simulink model "simulation_environment"  (R2018b)
settings: Solver=VariableStepAuto  StartTime=0.0  StopTime=50  RelTol=1e-3
libraries: follow_the_leader_library x3
settings Model: Creator=martin  LastModifiedBy=martin

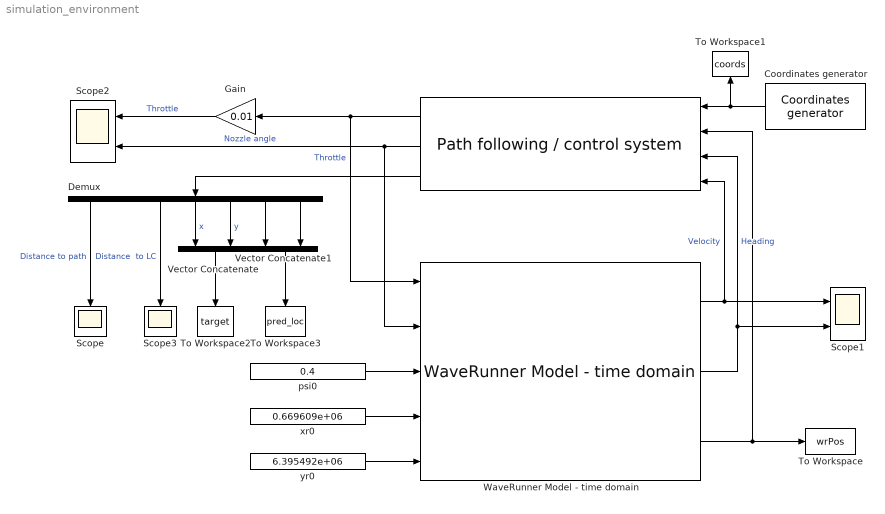
== system simulation_environment ==
  " " : follow_the_leader_library/Path following // control system  dt=2  g_Kp=4  g_Tf=5  g_Kd=0  g_Ki=5  g_max=100  g_min=0  n_Kp=-1  n_Tf=1  n_Kd=-100  n_Ki=0  n_max=18 * pi / 180  n_min=-18 * pi / 180
      settings: SourceProductName=Follow the leader
  Coordinates generator : follow_the_leader_library/Coordinates generator  fname=test3.txt  steptime=0.25
      settings: SourceProductName=Follow the leader
  Demux : Demux  Outputs=7
  Gain : Gain  Gain=0.01
  Scope : Scope
  Scope1 : Scope  NumInputPorts=2
  Scope2 : Scope  NumInputPorts=2
  Scope3 : Scope
  To Workspace : ToWorkspace  VariableName=wrPos  SaveFormat=Timeseries  SampleTime=0.1
  To Workspace1 : ToWorkspace  VariableName=coords  SaveFormat=Timeseries  SampleTime=-1
  To Workspace2 : ToWorkspace  VariableName=target  SaveFormat=Timeseries  SampleTime=0.1
      settings: Save2DSignal=2-D array (concatenate along first dimension)
  To Workspace3 : ToWorkspace  VariableName=pred_loc  SaveFormat=Timeseries  SampleTime=-1
  Vector Concatenate : Concatenate
  Vector Concatenate1 : Concatenate
  WaveRunner Model - time domain : follow_the_leader_library/WaveRunner Model - time domain  SystemSampleTime=-1
      link override Subsystem 3: Equation of Motion/Gain: Gain=8
      link override XY Graph: xmin=710332.2770471  xmax=710532.2770471  ymin=76269159.727303  ymax=76269359.727303
      settings: SourceProductName=Follow the leader
  psi0 : Constant  Value=0.4
  xr0 : Constant  Value=0.669609e+06
  yr0 : Constant  Value=6.395492e+06
  wires:
  WaveRunner Model - time domain/3 -> " "/2, To Workspace/1
  WaveRunner Model - time domain/2 -> " "/3, Scope1/2  "Heading"
  WaveRunner Model - time domain/1 -> " "/4, Scope1/1  "Velocity"
  psi0/1 -> WaveRunner Model - time domain/3
  xr0/1 -> WaveRunner Model - time domain/4
  yr0/1 -> WaveRunner Model - time domain/5
  Coordinates generator/1 -> " "/1, To Workspace1/1
  " "/3 -> Demux/1
  Demux/3 -> Scope3/1  "Distance  to LC"
  Vector Concatenate/1 -> To Workspace2/1
  Demux/4 -> Vector Concatenate/1  "x"
  Demux/5 -> Vector Concatenate/2  "y"
  Demux/6 -> Vector Concatenate1/1
  Demux/7 -> Vector Concatenate1/2
  Vector Concatenate1/1 -> To Workspace3/1
  " "/2 -> WaveRunner Model - time domain/2, Scope2/2  "Nozzle angle"
  Demux/1 -> Scope/1  "Distance to path"
  Gain/1 -> Scope2/1  "Throttle"
  " "/1 -> Gain/1, WaveRunner Model - time domain/1  "Throttle"
